simulink model "Switch_mod"  (R2020a)
settings: Solver=VariableStepAuto  StartTime=0.0  StopTime=10.0  RelTol=1e-3
libraries: autolibshared x1
settings Model: DataDictionary=Data_diction.sldd  Creator=ASD  LastModifiedBy=44689

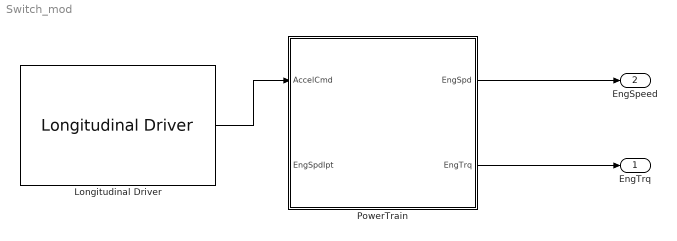
== system Switch_mod ==
  Longitudinal Driver : autolibshared/Longitudinal Driver  extAccelOvr=off  extDecelOvr=off  extAccelHld=off  extDecelHld=off  extAccelZero=off  extDecelZero=off  cntrlType=PI  shftType=None  velUnits=m/s  gearOut=off  Kp=15  Ki=1  Kff=.05  Kg=.01  VehVelVec=[0 100]  KffVec=[.1 .1]  KpVec=[10 10]  KiVec=[5 5]  KgVec=[0 0]  m=1500  Kpt=3000  tau=.1  L=2  aR=200  bR=2.5  cR=.5  g=9.81  vnom=100  Kaw=.1  tauerr=.03  tauPt=2  GearInit=0  tShift=.1  pdlVec=[0.1 0.4 0.5 0.9]  upShftTbl=[-1 12.9375 26.4375 39.9375 51.18749999999999 62.4375 72.84375 83.25;-1 16.3125 29.8125 43.3125 54.5624 65.8125 76.78125 87.75;-1 19.6875 33.1875 46.68749999999999 57.9375 69.1875 80.71875 92.25;-1 33 52.5 77.25 100.5 138.75 161.875 185]  dwnShftTbl=[1 9.5625 23.0625 36.5625 47.8125 59.0625 68.90625 78.75;1 12.9375 26.4375 39.9375 51.18749999999999 62.4375 72.84375 83.25;1 16.3125 29.8125 43.3125 54.562499 65.8125 76.78125 87.75;1 19.6875 33.1875 46.68749999999999 57.9375 69.1875 80.71875 92.25]  tClutch=.5  tRev=.5  tPark=120  aMode=1  UpGearVec="[0  1  2  3  4  5  6  7]"  DownGearVec="[1  2  3  4  5  6  7  8]"
      settings: SourceProductBaseCode=PW,MT,VE,VP
  PowerTrain : Subsystem  Variant=on
  EngTrq : Outport
  EngSpeed : Outport  Port=2
  wires:
  PowerTrain/2(EngTrq) -> EngTrq/1
  Longitudinal Driver/2 -> PowerTrain/1(AccelCmd)
  PowerTrain/1(EngSpd) -> EngSpeed/1

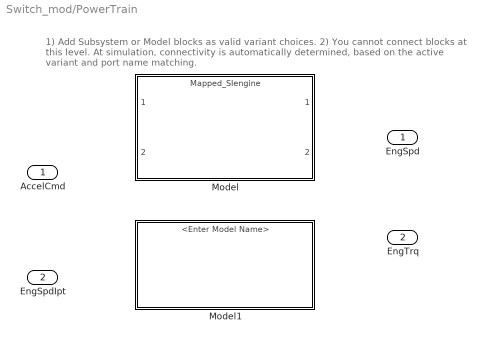
== system Switch_mod/PowerTrain ==
  note: 1) Add Subsystem or Model blocks as valid variant choices.
      | 2) You cannot connect blocks at this level. At simulation, connectivity is automatically
      | determined, based on the active variant and port name matching.
  AccelCmd : Inport
  EngSpdIpt : Inport  Port=2
  Model : ModelReference  DisableCoverage=on  ModelNameDialog=Mapped_SIengine.slx  VariantControl=pwrSwitch == 1  ModelReferenceVersion=1.17
  Model1 : ModelReference  VariantControl=pwrSwitch == 2
  EngSpd : Outport
  EngTrq : Outport  Port=2
